simulink model "mOvertakeManeuver"  (R2018b)
settings: Solver=VariableStepAuto  StartTime=0.0  StopTime=simTime  RelTol=1e-3
PreLoadFcn:
  | load 'tableStructure.mat'
InitFcn:
  | modelParams
  | clear markedSmartActorCount;
values from neighbouring files (symbols this model uses):
  initYPos = (scene.RoadNetwork.RoadCenters(1, 2) - laneWidth / 2)    [modelParams.m]
  initYPosRogue = (scene.RoadNetwork.RoadCenters(1, 2) - laneWidth / 2)    [modelParams.m]
  laneWidth = roadWidth / (scene.RoadNetwork.NumMarkings - 1)    [modelParams.m]
  maxLanes = 10    [modelParams.m]
  maxVehicles = 25    [modelParams.m]
  minOvertakeProximity = 50    [modelParams.m]
  numActors = length(scene.vehiclePoses(1).ActorPoses)    [modelParams.m]    (also in sessionLogReader.m = numel(inStruct); visualizer.m = numel(actors))
  numAddedRogueActors = 0    [modelParams.m]
  numLanes = scene.RoadNetwork.NumLanes    [modelParams.m]    (also in sessionLogReader.m = numMarkings-1)
  numSmartActors = 0    [modelParams.m]
  numSmartActorsDM = 0    [modelParams.m]
  rogueActorIdBase = 4000    [modelParams.m]
  safeTimeGap = 1.4    [modelParams.m]
  sensorRange = 600    [modelParams.m]
  smartActors = 0    [modelParams.m]    (also in sessionLogReader.m = repmat(actorPoses(1), [obj.NumSmartActors, 1]))
  smartActorsDM = 0    [modelParams.m]    (also in sessionLogReader.m = repmat(actorPoses(1), [obj.NumSmartActorsDM, 1]))
  standStillGap = 10    [modelParams.m]
  W_SPEC = [Ln1;vdes;vmax;AXadd;AXmult;BXadd;BXmult;EXadd;EXmult;CXconst;CXadd;CXmult;OPDVmult;OPDVadd;BNULLmult;BMAXmult;FAKTORVmult;BMINadd;BMINmult;      RND1n;RND2n;RND3n;RND4n;NRND]    [wiedemannParams.m]
undefined symbols (not defined in the file or in its folder): actorPoseInit, addedRogueVelocity, addedRogueXPosition, DiscIntNeverNeededParam
libraries: dataTableBlockslib x2, mpcadaslib x1
(part 1 of 3)
settings Model: Creator=surongal  LastModifiedBy=surongal
settings DataIOCC: SaveTime=off  ReturnWorkspaceOutputs=on
settings DebuggingCC: InheritedTsInSrcMsg=none
settings SFSimCC: SimUseLocalCustomCode=off
settings RTWCC: RTWUseLocalCustomCode=off

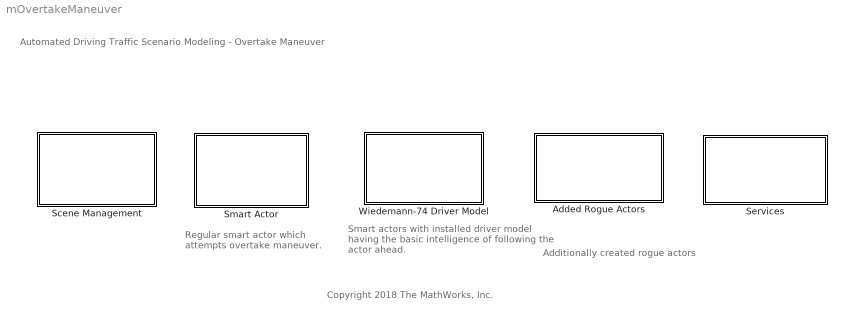
== system mOvertakeManeuver ==
  note: Smart actors with installed driver model having the basic intelligence of following the actor ahead.
  note: Regular smart actor which attempts overtake maneuver.
  note: Copyright 2018 The MathWorks, Inc.
  note: Automated Driving Traffic Scenario Modeling - Overtake Maneuver
  note: Additionally created rogue actors
  Added Rogue Actors : Subsystem  InitFcn=|  mask(Added Rogue Actors){numAddedRogueCars=2, initXPos=[5 550], initXVel=[5 10], rogueActorIdBase=4000}
      | % To get the mask parameter values
      | numAddedRogueActors =str2num( get_param(gcb,'numAddedRogueCars'));
      | addedRogueXPosition = str2num( get_param(gcb,'initXPos'));
      | addedRogueVelocity = str2num( get_param(gcb,'initXVel'));
      | 
      | % To set the mask parameter values
      | set_param(gcb, 'rogueActorIdBase',num2str(rogueActorIdBase));
      mask prompts: numAddedRogueCars "Number of rogue actors"; initXPos "Initial X-position"; initXVel "Initial X-velocity"
      mask help: This block allows to introduce additional rogue actors to the scenario. Each parameter array sequentially contains parameter value for different actors. The scenario should contain only one rogue actors block.
      mask Display:
      | numRogueActors = str2num(get_param(gcb,'numAddedRogueCars'));
      | rogueActorIdBase = str2num(get_param(gcb,'rogueActorIdBase'));
      | disp("Actor IDs : [" + num2str(rogueActorIdBase + [1:numRogueActors]) + "]");
  Scene Management : Subsystem
      mask Display: disp('Scene Management')
  Services : Subsystem
      mask Display: disp('Services');
  Smart Actor : Subsystem  InitFcn=|  mask(Smart Actor){smartActorId=1, aggressivenessLevel=1, maxVelocity=20, maxAcceleration=3, maxDeceleration=-6}
      | smartActorId = str2num(get_param(gcb, 'smartActorId'));
      | % Update the number of actors marked as smart
      | numSmartActors = markedSmartActorCount();
      | 
      | % To keep track of marked smart actors
      | if ismember(smartActorId, smartActors)
      |     error('Actor ID specified is already marked as smart. Mark some other actor ID as smart');
      | else
      |     % To check actorId specified is present or not
      |     if ismember(smartActorId, [actorPoseInit.ActorID])
      |         smartActors(numSmartActors) = smartActorId;
      |     else
      |         error('Actor ID specified in Smart Actor does not exist.');
      |     end
      | end
      | 
      | % To check whether actorId specified as Smart is not already
      | % specified as a smart-actor with driver-model. 
      | driverModelBlockPath = [bdroot, '/Wiedemann-74 Driver Model'];
      | if getSimulinkBlockHandle(driverModelBlockPath) > 0
      |     if strcmp(get_param(driverModelBlockPath, 'commented'), 'off')
      |         % Get Actor IDs with driver model installed
      |         smartIdsDM = str2num(get_param(driverModelBlockPath, 'smartVehIdsDM'));
      |         if sum(ismember(smartActorId, smartIdsDM))
      |             error(['Driver model installation on Smart Actor ' num2str(smartActorId) ' is not supported.']);
      |         end
      |     end
      | end
      | 
      | clear driverModelBlockPath smartIdsDM smartActorId; % clear temporary variables
      mask prompts: smartActorId "ActorID"; aggressivenessLevel "Driver aggressiveness level"; maxVelocity "Max velocity"; maxAcceleration "Max acceleration"; maxDeceleration "Max deceleration"
      mask help: This block allows to mark an actor in the simulation log as a smart actor attempting overtake-maneuver.
      mask init:
      | aggressivenessLevel = str2num(aggressivenessLevel);
      | 
      | % To check whether actorId specified is already
      | % specified in the driver model
      | driverModelBlockPath = [bdroot, '/Wiedemann-74 Driver Model'];
      | if getSimulinkBlockHandle(driverModelBlockPath) > 0
      |     if strcmp(get_param(driverModelBlockPath, 'commented'), 'off')
      |         % Get smart actors with driver model installed
      |         smartIdsDM = str2num(get_param(driverModelBlockPath, 'smartVehIdsDM'));
      |         if sum(ismember(smartActorId, smartIdsDM))
      |             error(['Driver model is already installed on actor with Actor ID : ' num2str(smartActorId) '.']);
      |         end
      |     end
      | end
      mask TypeOptions aggressivenessLevel: 1 | 2 | 3
      mask Display: image('icons/car.png');
  Wiedemann-74 Driver Model : Subsystem  InitFcn=|  mask(Wiedemann-74 Driver Model){smartVehIdsDM=[2], AXAdd=[5], BXMult=[5], vMax=[40], vDes=[30], maxAccel=[4], maxDecel=[-6]}
      | smartActorsDM = str2num( get_param(gcb, 'smartVehIdsDM')); % IDs of vehicles with Driver-Model installed
      | numSmartActorsDM = length(smartActorsDM); % Number of vehicles with Driver-Model installed
      | 
      | wiedemannParams; % Loads Wiedemann model parameters
      | 
      | % All the actors IDs specified for driver-model installation are valid or not
      | if sum(ismember(smartActorsDM, [actorPoseInit.ActorID])) < numSmartActorsDM
      |     error(['Actor IDs [' num2str(smartActorsDM(~ismember(smartActorsDM, [actorPoseInit.ActorID]))) '] specified for driver-model installation does not exist.']);
      | end
      mask prompts: smartVehIdsDM "Vehicles with driver-model"; AXAdd "AXadd (Calibrated parameter affecting desired following distance between stationary vehicles)"; BXMult "BXmult (Calibrated parameter affecting desired minimum following distance at low speed gap)"; vMax "Maximum velocity"; vDes "Desired velocity"; maxAccel "Max acceleration"; maxDecel "Max deceleration"
      mask help: This block allows to install Wiedemann-74 car-follow model on the selected actors. Also, Widemann-74 driver model parameters can be configured for individual cars. Each parameter vector sequentially contains parameter value for different actors in same order as actors are specified in the vehicle's list.
      mask DialogControl maskInfo Prompt: Driver-Model Setup Table
      mask Display: image('icons/carFollow.png');

== system mOvertakeManeuver/Added Rogue Actors ==
  note: Create a set of rogue actors and simulate their movement
  note: Rogue Actors
  "Calculate updated X-Poses " : Subsystem  TreatAsAtomicUnit=on
  Calculate updated Y-Poses : Subsystem  TreatAsAtomicUnit=on
  Get initial poses : MATLAB Function  TreatAsAtomicUnit=on
  Publish to data-table : MATLAB Function  TreatAsAtomicUnit=on
  wires:
  "Calculate updated X-Poses "/2(posVector) -> Publish to data-table/2(xPosVector)
  "Calculate updated X-Poses "/1(velVector) -> Publish to data-table/1(xVelVector)
  Get initial poses/5(yVelocity) -> Calculate updated Y-Poses/2(initVelVector)
  Get initial poses/6(yPosition) -> Calculate updated Y-Poses/3(initPosVector)
  Get initial poses/4(yAcceleration) -> Calculate updated Y-Poses/1(accelVector)
  Calculate updated Y-Poses/1(velVector) -> Publish to data-table/3(yVelVector)
  Calculate updated Y-Poses/2(posVector) -> Publish to data-table/4(yPosVector)
  Get initial poses/1(xAcceleration) -> "Calculate updated X-Poses "/1(accelVector)
  Get initial poses/2(xVelocity) -> "Calculate updated X-Poses "/2(initVelVector)
  Get initial poses/3(xPosition) -> "Calculate updated X-Poses "/3(initPosVector)

== system mOvertakeManeuver/Scene Management ==
  Actor Pose Reader : Subsystem  mask(Actor Pose Reader){ScenarioFileName=scenarioInput, RoadBoundaries=on, LaneBoundaries=on, AllBoundaries=on, LaneMarkings=on, NumLanes=off, NumSmartActorsDM=numSmartActorsDM, NumSmartActors=numSmartActors}
      mask prompts: ScenarioFileName "File name for the recorded scenario:"; RoadBoundaries "Output road boundaries in scenario coordinates"; LaneBoundaries "Output lane boundaries in scenario coordinates"; AllBoundaries "Output all lane boundaries"; LaneMarkings "Output lane markings in scenario coordinates"; NumLanes "Output number of lanes"; NumSmartActorsDM "Number of actors with driver model installed:"; NumSmartActors "Number of actors marked as smart:"
      mask help: The Actor Pose Reader reads actor poses data saved using the drivingScenario record method and road boundary data saved as structs from the drivingScenario roadBoundaries method.
      mask TypeOptions ScenarioFileName: Session Log Reader/ScenarioFileName
      mask TypeOptions RoadBoundaries: Session Log Reader/RoadBoundaries
      mask TypeOptions LaneBoundaries: Session Log Reader/LaneBoundaries
      mask TypeOptions AllBoundaries: Session Log Reader/AllBoundaries
      mask TypeOptions LaneMarkings: Session Log Reader/LaneMarkings
      mask TypeOptions NumLanes: Session Log Reader/NumLanes
      mask TypeOptions NumSmartActorsDM: Session Log Reader/NumSmartActorsDM
      mask TypeOptions NumSmartActors: Session Log Reader/NumSmartActors
      mask Display:
      | disp(['Session Log' char(10) 'Reader']);
      | port_label('output',1,'Actors');
      | port_label('output',2,'Lane Boundaries');
      | port_label('output',3,'Roads');
      | port_label('output',4,'Lane Markings');
  Append poses of added rouge actors for visualization : Subsystem  InitFcn=""
  Publish To Data Table : Subsystem  InitFcn=""
  Visualization : Subsystem  mask(Visualization){XLim=[ -1, 150 ], YLim=[ -30, 30 ], View=Self-Centered view, NumSmartActors=numSmartActors, HasActors=on, HasRoads=on, HasLaneMarkings=on}
      mask prompts: XLim "Minimum and maximum distance in the longitudinal axis:"; YLim "Minimum and maximum distance in the lateral axis:"; View "Visualization type:"; NumSmartActors "Number of smart actors:"; HasActors "Display actors data"; HasRoads "Display road boundary data"; HasLaneMarkings "Display lane markings"
      mask help: The Visualization block creates and maintains a bird's-eye plot. You can opt for 'World-coordinate' view or 'Self-centered' view.
      mask TypeOptions XLim: Visualization/XLim
      mask TypeOptions YLim: Visualization/YLim
      mask TypeOptions View: Visualization/View
      mask TypeOptions NumSmartActors: Visualization/NumSmartActors
      mask TypeOptions HasActors: Visualization/HasActors
      mask TypeOptions HasRoads: Visualization/HasRoads
      mask TypeOptions HasLaneMarkings: Visualization/HasLaneMarkings
      mask Display:
      | disp('Visualizer');
      | port_label('input',1,'Actors');
      | port_label('input',2,'Roads');
      | port_label('input',3,'Lane Markings');
  wires:
  Actor Pose Reader/3(Roads) -> Visualization/2(Roads)
  Actor Pose Reader/1(Actors) -> Publish To Data Table/1(Actors), Append poses of added rouge actors for visualization/1(simulationLogActors)
  Actor Pose Reader/2(Lane Boundaries) -> Publish To Data Table/2(Lane Boundaries)
  Actor Pose Reader/4(Lane Markings) -> Visualization/3(Lane Markings)
  Append poses of added rouge actors for visualization/1(actors) -> Visualization/1(Actors)  "actorPoses"

== system mOvertakeManeuver/Services ==
  note: Queries used by Smart Agents
  "Actor-Pose " : dataTableBlockslib/Data Table Service  tableName=Actor  tableSize=30  tableFormat=Vehicle  tableQueries={{OvertakeQueries.VehiclesAheadSameLane,'findVehiclesAheadSameLane'},{OvertakeQueries.VehiclesAheadLeftLane,'findVehiclesAheadLeftLane'}}  mask(DataTableService){}
      mask Display: disp('Actor Pose Information');
  Find approaching vehicles in the left lane : Subsystem  TreatAsAtomicUnit=on
  Find vehicles ahead in the same lane : Subsystem  TreatAsAtomicUnit=on
  Global to self-centered pose conversion : Subsystem  TreatAsAtomicUnit=on
  "Scene " : dataTableBlockslib/Data Table Service  tableName=Scenario  tableSize=30  tableFormat=LaneBoundaries  tableQueries={}  mask(DataTableService){}
      mask Display: disp('Scene Information');

== system mOvertakeManeuver/Smart Actor ==
  note: This subsystem simulates an actor which is nominated as a smart actor,
      | among the actors present in input driving session log. The primary intelligence in this
      | smart actor is to overtake, if environment around it allows for it.
  note: Nominated Smart Actor
  Load Initial Pose : MATLAB Function  TreatAsAtomicUnit=on
  Smart Actor system : Subsystem
  Write pose to Data-Table : MATLAB Function  TreatAsAtomicUnit=on
  wires:
  Smart Actor system/1(Updated Pose) -> Write pose to Data-Table/1(pose)
  Load Initial Pose/1(initPose) -> Smart Actor system/1(Initial Pose)

== system mOvertakeManeuver/Wiedemann-74 Driver Model ==
  note: Apply driver-model on selected actors:
      | Calculated updated driver-model-governed poses and write into data-table.
  Apply driver-model : Subsystem
  Get Follow and Lead car : MATLAB Function  TreatAsAtomicUnit=on
  Gets the vehicles ahead in sorted order of the distance from this actor. : Subsystem  TreatAsAtomicUnit=on
  Simulation Time : DigitalClock  SampleTime=-1
  Write smart-actor poses in data-table : MATLAB Function  TreatAsAtomicUnit=on
  wires:
  Apply driver-model/1(velVector) -> Write smart-actor poses in data-table/1(velVector)
  Get Follow and Lead car/5(leadAcc) -> Apply driver-model/5(leadVehAcc)
  Get Follow and Lead car/4(leadVel) -> Apply driver-model/4(leadVehSpd)
  Apply driver-model/2(posVector) -> Write smart-actor poses in data-table/2(posVector)
  Get Follow and Lead car/2(follVel) -> Apply driver-model/2(smartVehSpd)
  Simulation Time/1 -> Get Follow and Lead car/1(timestamp)
  Get Follow and Lead car/1(follPos) -> Apply driver-model/1(smartVehPos)
  Get Follow and Lead car/3(leadPos) -> Apply driver-model/3(leadVehPos)

== system mOvertakeManeuver/Added Rogue Actors/Calculate updated X-Poses  ==
  accelVector : Inport  Partition=on  PartitionDimension=1  PartitionWidth=1  PartitionOffset=0
  initVelVector : Inport  Port=2  Partition=on  PartitionDimension=1  PartitionWidth=1  PartitionOffset=0
  initPosVector : Inport  Port=3  Partition=on  PartitionDimension=1  PartitionWidth=1  PartitionOffset=0
  For Each : ForEach  DisableCoverage=on  IndexMode=One-based
  Update Poses : Subsystem
  velVector : Outport  ConcatenationDimension=1
  posVector : Outport  Port=2  ConcatenationDimension=1
  wires:
  accelVector/1 -> Update Poses/1(accVector)
  initPosVector/1 -> Update Poses/3(initPosVector)
  initVelVector/1 -> Update Poses/2(initVelVector)
  Update Poses/2(Out2) -> posVector/1
  Update Poses/1(Out1) -> velVector/1

== system mOvertakeManeuver/Added Rogue Actors/Calculate updated Y-Poses ==
  accelVector : Inport  Partition=on  PartitionDimension=1  PartitionWidth=1  PartitionOffset=0
  initVelVector : Inport  Port=2  Partition=on  PartitionDimension=1  PartitionWidth=1  PartitionOffset=0
  initPosVector : Inport  Port=3  Partition=on  PartitionDimension=1  PartitionWidth=1  PartitionOffset=0
  For Each : ForEach  DisableCoverage=on  IndexMode=One-based
  Update Poses : Subsystem
  velVector : Outport  ConcatenationDimension=1
  posVector : Outport  Port=2  ConcatenationDimension=1
  wires:
  Update Poses/1(Out1) -> velVector/1
  Update Poses/2(Out2) -> posVector/1
  initVelVector/1 -> Update Poses/2(initVelVector)
  initPosVector/1 -> Update Poses/3(initPosVector)
  accelVector/1 -> Update Poses/1(accVector)

== system mOvertakeManeuver/Scene Management/Actor Pose Reader ==
  Read smart actor poses : MATLAB Function  TreatAsAtomicUnit=on
  Session Log Reader : MATLABSystem  System=sessionLogReader  ScenarioFileName=scenarioInput  NumSmartActorsDM=NumSmartActorsDM  NumSmartActors=NumSmartActors  SmartActorSource=Input port  SmartActorID=1  RoadBoundaries=on  LaneBoundaries=on  AllBoundaries=on  LaneBoundaryDistance=0:0.5:9.5  LaneBoundaryLocation=center  NumLanes=off  LaneMarkings=on  BusNameSource=Auto  BusName2Source=Auto  BusName3Source=Auto  SimulateUsing=Interpreted execution
      mask Type: sessionLogReader
      mask Display:
      | disp(['Session Log' char(10) 'Reader']);
      | port_label('input',1,'actors');
      | port_label('output',1,'Actors');
      | port_label('output',2,'Roads');
      | port_label('output',3,'Lane Boundaries');
      | port_label('output',4,'Lane Markings');
  Actors : Outport
  Lane Boundaries : Outport  Port=2
  Roads : Outport  Port=3
  Lane Markings : Outport  Port=4
  wires:
  Session Log Reader/1 -> Actors/1
  Session Log Reader/2 -> Roads/1
  Session Log Reader/4 -> Lane Markings/1
  Session Log Reader/3 -> Lane Boundaries/1
  Read smart actor poses/1(actorPoses) -> Session Log Reader/1

== system mOvertakeManeuver/Scene Management/Append poses of added rouge actors for visualization ==
  simulationLogActors : Inport
  Appending Rouge Actor Poses : MATLAB Function  TreatAsAtomicUnit=on
  Bus Selector1 : BusSelector  OutputSignals=Actors
  actors : Outport
  wires:
  Bus Selector1/1 -> Appending Rouge Actor Poses/1(simulationLogActors)  "<Actors>"
  simulationLogActors/1 -> Bus Selector1/1
  Appending Rouge Actor Poses/1(Actors) -> actors/1

== system mOvertakeManeuver/Scene Management/Publish To Data Table ==
  Actors : Inport
  Lane Boundaries : Inport  Port=2
  Bus Selector : BusSelector  OutputSignals=Actors
  Write inital pose from session-logs into data-table : MATLAB Function  Priority=0  TreatAsAtomicUnit=on
      settings: AttributesFormatString=Pri = %<Priority>
  update data tables : MATLAB Function  TreatAsAtomicUnit=on
  wires:
  Actors/1 -> Bus Selector/1
  Bus Selector/1 -> update data tables/1(actors)  "<Actors>"
  Lane Boundaries/1 -> update data tables/2(laneBoundaryInfo)

== system mOvertakeManeuver/Scene Management/Visualization ==
  Actors : Inport
  Roads : Inport  Port=2
  Lane Markings : Inport  Port=3
  Visualization : MATLABSystem  StartFcn=|  StopFcn=""  System=visualizer  XLim=XLim  YLim=YLim  NumSmartActors=NumSmartActors  View=Self-Centered view  smartActorIndex=1  HasActors=on  HasRoads=on  HasLaneMarkings=on
      | % checks whether the view is set to Ego Centric View
      | if strcmp(get_param(gcb, 'View'), 'Self-Centered view')
      |     % checks whether to populate the list modal dialog
      |     if numSmartActors > 1
      |         List = repmat("Added Ego (Actor ID : ", [numSmartActors 1]);
      |         for n = 1 : numSmartActors
      |             List(n, 1) =   "Nominated Ego  (Actor ID : "+smartActors(n)+")";
      |         end
      |         
      |         [indx, isSelected] = listdlg('PromptString', 'Select the ego actor ', 'ListString', List, 'SelectionMode', 'single', 'InitialValue', 1);
      |         % if user closes the dialog without selecting from list
      |         if isSelected == 0
      |             % set the indx to 1
      |             indx = 1;
      |         end
      |     else
      |         indx = 1;
      |     end
      |     
      |     % Set the mask parameters
      |     set_param(gcb, 'smartActorIndex', num2str(indx));
      | end
      | 
      | clear List n indx isSelected; % clears temporary variables
      mask Type: visualizer
      mask Display:
      | disp('Visualizer');
      | port_label('input',1,'Actors');
      | port_label('input',2,'Roads');
      | port_label('input',3,'Lane Markings');
  wires:
  Roads/1 -> Visualization/2
  Lane Markings/1 -> Visualization/3
  Actors/1 -> Visualization/1

== system mOvertakeManeuver/Services/Find approaching vehicles in the left lane ==
  findVehiclesAheadLeftLane : TriggerPort  TriggerType=function-call  IsSimulinkFunction=on  FunctionName=findVehiclesAheadLeftLane  FunctionVisibility=scoped  VariantControl=(inherit)
  MATLAB Function : MATLAB Function  TreatAsAtomicUnit=on
  refEntry : ArgIn  OutDataTypeStr=Bus: Vehicle  ArgumentName=refEntry
  otherEntry : ArgIn  Port=2  OutDataTypeStr=Bus: Vehicle  ArgumentName=otherEntry
  matched : ArgOut  DisableCoverage=on  OutDataTypeStr=boolean  ArgumentName=matched
  wires:
  MATLAB Function/1(matched) -> matched/1
  refEntry/1 -> MATLAB Function/1(refPose)
  otherEntry/1 -> MATLAB Function/2(candidatePose)

== system mOvertakeManeuver/Services/Find vehicles ahead in the same lane ==
  findVehiclesAheadSameLane : TriggerPort  TriggerType=function-call  IsSimulinkFunction=on  FunctionName=findVehiclesAheadSameLane  FunctionVisibility=scoped  VariantControl=(inherit)
  MATLAB Function : MATLAB Function  TreatAsAtomicUnit=on
  refEntry : ArgIn  OutDataTypeStr=Bus: Vehicle  ArgumentName=refEntry
  otherEntry : ArgIn  Port=2  OutDataTypeStr=Bus: Vehicle  ArgumentName=otherEntry
  matched : ArgOut  DisableCoverage=on  OutDataTypeStr=boolean  ArgumentName=matched
  wires:
  MATLAB Function/1(matched) -> matched/1
  refEntry/1 -> MATLAB Function/1(refPose)
  otherEntry/1 -> MATLAB Function/2(candidatePose)

== system mOvertakeManeuver/Services/Global to self-centered pose conversion ==
  globalToSelfCentered : TriggerPort  TriggerType=function-call  IsSimulinkFunction=on  FunctionName=globalToSelfCentered  VariantControl=(inherit)
  Self-Centered Pose Conversion : MATLAB Function  TreatAsAtomicUnit=on
  refEntry : ArgIn  DisableCoverage=on  OutDataTypeStr=Bus: Vehicle  ArgumentName=refEntry
  otherEntry : ArgIn  Port=2  OutDataTypeStr=Bus: Vehicle  ArgumentName=otherEntry
  selfRefInfo : ArgOut  DisableCoverage=on  OutDataTypeStr=Bus: Vehicle  ArgumentName=selfRefInfo
  wires:
  refEntry/1 -> Self-Centered Pose Conversion/1(selfPose)
  otherEntry/1 -> Self-Centered Pose Conversion/2(otherVehPose)
  Self-Centered Pose Conversion/1(egoCentricInfo) -> selfRefInfo/1

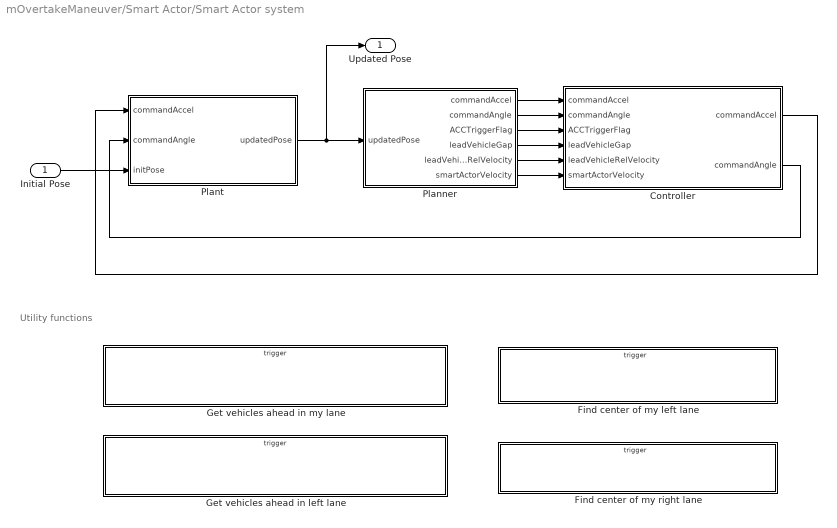
== system mOvertakeManeuver/Smart Actor/Smart Actor system ==
  note: Utility functions
  Initial Pose : Inport
  Controller : Subsystem
  Find center of my left lane : Subsystem  TreatAsAtomicUnit=on
  Find center of my right lane : Subsystem  TreatAsAtomicUnit=on
  Get vehicles ahead in left lane : Subsystem  TreatAsAtomicUnit=on
  Get vehicles ahead in my lane : Subsystem  TreatAsAtomicUnit=on
  Planner : Subsystem
  Plant : Subsystem
  Updated Pose : Outport
  wires:
  Initial Pose/1 -> Plant/3(initPose)
  Controller/1(commandAccel) -> Plant/1(" commandAccel")
  Plant/1(updatedPose) -> Planner/1(updatedPose), Updated Pose/1
  Planner/1(commandAccel) -> Controller/1(" commandAccel")
  Planner/2(commandAngle) -> Controller/2(" commandAngle")
  Planner/3(ACCTriggerFlag) -> Controller/3(ACCTriggerFlag)
  Planner/4(leadVehicleGap) -> Controller/4(" leadVehicleGap")
  Planner/5(leadVehicleRelVelocity) -> Controller/5(" leadVehicleRelVelocity")
  Planner/6(smartActorVelocity) -> Controller/6(" smartActorVelocity")
  Controller/2(commandAngle) -> Plant/2(commandAngle)

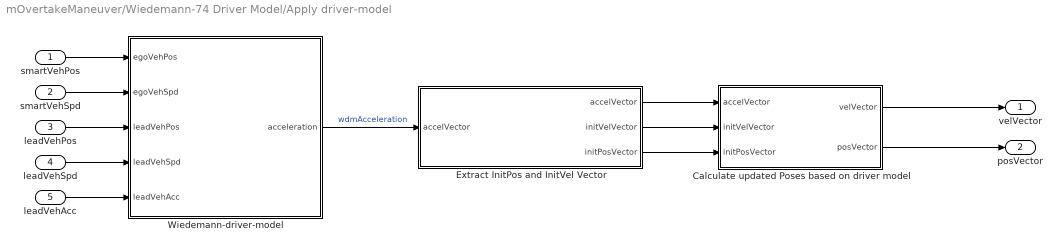
== system mOvertakeManeuver/Wiedemann-74 Driver Model/Apply driver-model ==
  smartVehPos : Inport
  smartVehSpd : Inport  Port=2
  leadVehPos : Inport  Port=3
  leadVehSpd : Inport  Port=4
  leadVehAcc : Inport  Port=5
  Calculate updated Poses based on driver model : Subsystem  TreatAsAtomicUnit=on
  Extract InitPos and InitVel Vector : MATLAB Function  TreatAsAtomicUnit=on
  Wiedemann-driver-model : Subsystem
  velVector : Outport
  posVector : Outport  Port=2
  wires:
  smartVehPos/1 -> Wiedemann-driver-model/1(egoVehPos)
  smartVehSpd/1 -> Wiedemann-driver-model/2(egoVehSpd)
  leadVehPos/1 -> Wiedemann-driver-model/3(leadVehPos)
  leadVehSpd/1 -> Wiedemann-driver-model/4(leadVehSpd)
  leadVehAcc/1 -> Wiedemann-driver-model/5(leadVehAcc)
  Calculate updated Poses based on driver model/1(velVector) -> velVector/1
  Calculate updated Poses based on driver model/2(posVector) -> posVector/1
  Extract InitPos and InitVel Vector/1(accelVector) -> Calculate updated Poses based on driver model/1(accelVector)
  Extract InitPos and InitVel Vector/3(initPosVector) -> Calculate updated Poses based on driver model/3(initPosVector)
  Extract InitPos and InitVel Vector/2(initVelVector) -> Calculate updated Poses based on driver model/2(initVelVector)
  Wiedemann-driver-model/1(acceleration) -> Extract InitPos and InitVel Vector/1("accelVector ")  "wdmAcceleration"

== system mOvertakeManeuver/Wiedemann-74 Driver Model/Gets the vehicles ahead in sorted order of the distance from this actor. ==
  getVehAheadSorted : TriggerPort  TriggerType=function-call  IsSimulinkFunction=on  FunctionName=getVehAheadSorted  FunctionVisibility=scoped  VariantControl=(inherit)
  Gets the vehicles ahead in sorted order of the gap : MATLAB Function  TreatAsAtomicUnit=on
  actorId : ArgIn  DisableCoverage=on  ArgumentName=actorId
  numVeh : ArgOut  ArgumentName=numVeh
  vehAheadInfo : ArgOut  Port=2  OutDataTypeStr=Bus: Vehicle  PortDimensions=maxVehicles  ArgumentName=vehAheadInfo
  wires:
  actorId/1 -> Gets the vehicles ahead in sorted order of the gap/1(actorId)
  Gets the vehicles ahead in sorted order of the gap/1(vehAheadInfo) -> vehAheadInfo/1
  Gets the vehicles ahead in sorted order of the gap/2(numVeh) -> numVeh/1

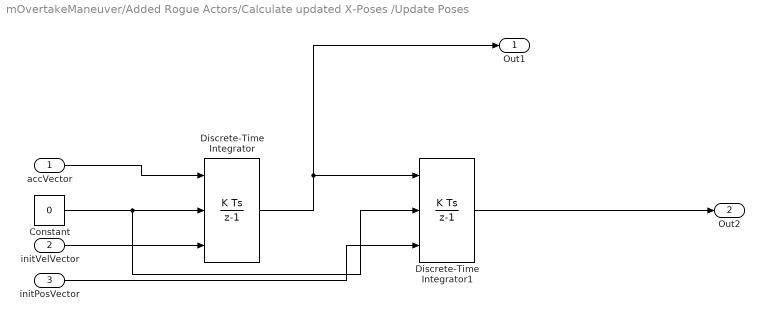
== system mOvertakeManeuver/Added Rogue Actors/Calculate updated X-Poses /Update Poses ==
  accVector : Inport
  initVelVector : Inport  Port=2
  initPosVector : Inport  Port=3
  Constant : Constant  Value=0
  Discrete-Time Integrator : DiscreteIntegrator  ExternalReset=level  InitialConditionSource=external  SampleTime=-1  ICPrevOutput=DiscIntNeverNeededParam  ICPrevScaledInput=DiscIntNeverNeededParam
  Discrete-Time Integrator1 : DiscreteIntegrator  ExternalReset=level  InitialConditionSource=external  SampleTime=-1  ICPrevOutput=DiscIntNeverNeededParam  ICPrevScaledInput=DiscIntNeverNeededParam
  Out1 : Outport
  Out2 : Outport  Port=2
  wires:
  Discrete-Time Integrator/1 -> Discrete-Time Integrator1/1, Out1/1
  accVector/1 -> Discrete-Time Integrator/1
  Discrete-Time Integrator1/1 -> Out2/1
  initPosVector/1 -> Discrete-Time Integrator1/3
  Constant/1 -> Discrete-Time Integrator1/2, Discrete-Time Integrator/2
  initVelVector/1 -> Discrete-Time Integrator/3

== system mOvertakeManeuver/Added Rogue Actors/Calculate updated Y-Poses/Update Poses ==
  accVector : Inport
  initVelVector : Inport  Port=2
  initPosVector : Inport  Port=3
  Constant : Constant  Value=0
  Discrete-Time Integrator : DiscreteIntegrator  ExternalReset=level  InitialConditionSource=external  SampleTime=-1  ICPrevOutput=DiscIntNeverNeededParam  ICPrevScaledInput=DiscIntNeverNeededParam
  Discrete-Time Integrator1 : DiscreteIntegrator  ExternalReset=level  InitialConditionSource=external  SampleTime=-1  ICPrevOutput=DiscIntNeverNeededParam  ICPrevScaledInput=DiscIntNeverNeededParam
  Out1 : Outport
  Out2 : Outport  Port=2
  wires:
  Constant/1 -> Discrete-Time Integrator1/2, Discrete-Time Integrator/2
  initPosVector/1 -> Discrete-Time Integrator1/3
  Discrete-Time Integrator1/1 -> Out2/1
  accVector/1 -> Discrete-Time Integrator/1
  initVelVector/1 -> Discrete-Time Integrator/3
  Discrete-Time Integrator/1 -> Discrete-Time Integrator1/1, Out1/1

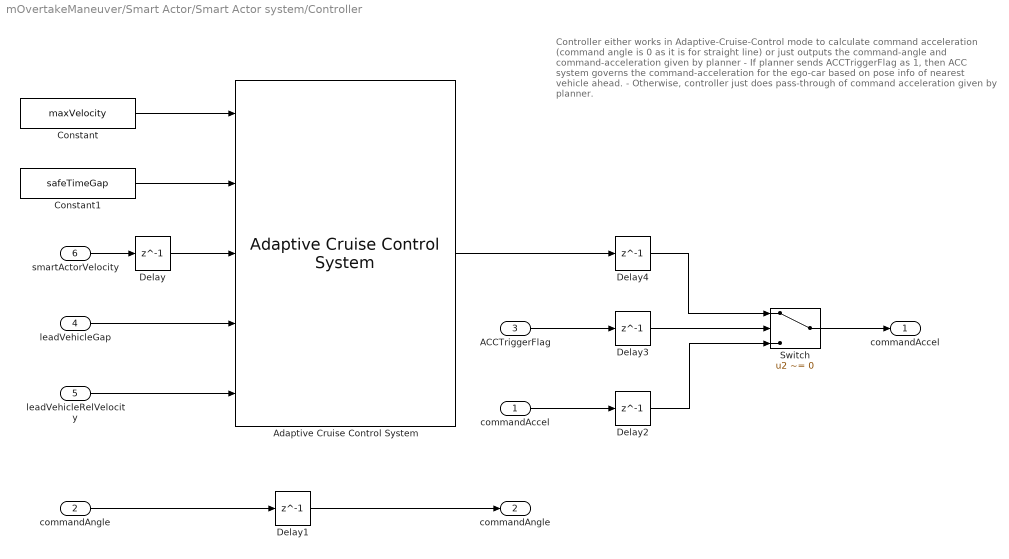
== system mOvertakeManeuver/Smart Actor/Smart Actor system/Controller ==
  note: Controller either works in Adaptive-Cruise-Control mode to calculate
      | command acceleration (command angle is 0 as it is for straight line) or
      | just outputs the command-angle and command-acceleration given by
      | planner
      | - If planner sends ACCTriggerFlag as 1, then ACC system governs the
      |   command-acceleration for the ego-car based on pose info
      |   of nearest vehicle ahead.
      | - Otherwise, controller just does pass-through of command acceleration
      |   given by planner.
  " commandAccel" : Inport
  " commandAngle" : Inport  Port=2
  ACCTriggerFlag : Inport  Port=3
  " leadVehicleGap" : Inport  Port=4
  " leadVehicleRelVelocity" : Inport  Port=5
  " smartActorVelocity" : Inport  Port=6
  Adaptive Cruise Control System : mpcadaslib/Adaptive Cruise Control System  EgoModel=tf(1,[0.5,1,0])  InitialEgoVelocity=abs(actorPoseInit(smartActorId).Velocity(1))  DefaultSpacing=standStillGap  MaxVelocity=maxVelocity  MinAcceleration=maxDeceleration  amin_ext=off  MaxAcceleration=maxAcceleration  amax_ext=off  Ts=0.1  PredictionHorizon=30  ControllerBehavior=0.5  suboptimal=off  maxiter=10  datatypeopt=double  optmode=off  trackmode=off
      settings: SourceProductName=Model Predictive Control Toolbox
  Constant : Constant  Value=maxVelocity  SampleTime=-1
  Constant1 : Constant  Value=safeTimeGap
  Delay{,1..4} (5 alike) : Delay  DelayLength=1  InitialCondition=0
  Switch : Switch  Criteria=u2 ~= 0
  commandAccel : Outport
  commandAngle : Outport  Port=2
  wires:
  " commandAccel"/1 -> Delay2/1
  Constant/1 -> Adaptive Cruise Control System/1
  " leadVehicleGap"/1 -> Adaptive Cruise Control System/4
  " leadVehicleRelVelocity"/1 -> Adaptive Cruise Control System/5
  " commandAngle"/1 -> Delay1/1
  Delay/1 -> Adaptive Cruise Control System/3
  Delay1/1 -> commandAngle/1
  " smartActorVelocity"/1 -> Delay/1
  ACCTriggerFlag/1 -> Delay3/1
  Delay2/1 -> Switch/3
  Delay3/1 -> Switch/2
  Delay4/1 -> Switch/1
  Adaptive Cruise Control System/1 -> Delay4/1
  Constant1/1 -> Adaptive Cruise Control System/2
  Switch/1 -> commandAccel/1

== system mOvertakeManeuver/Smart Actor/Smart Actor system/Find center of my left lane ==
  getLeftLane : TriggerPort  TriggerType=function-call  IsSimulinkFunction=on  FunctionName=getLeftLane  FunctionVisibility=scoped  VariantControl=(inherit)
  Get left lane center Y : MATLAB Function  TreatAsAtomicUnit=on
  currPose : ArgIn  OutDataTypeStr=Bus: Vehicle  ArgumentName=currPose
  leftLaneCenter : ArgOut  ArgumentName=leftLaneCenter
  wires:
  currPose/1 -> Get left lane center Y/1(currPose)
  Get left lane center Y/1(leftlaneY) -> leftLaneCenter/1

== system mOvertakeManeuver/Smart Actor/Smart Actor system/Find center of my right lane ==
  getRightLane : TriggerPort  TriggerType=function-call  IsSimulinkFunction=on  FunctionName=getRightLane  FunctionVisibility=scoped  VariantControl=(inherit)
  Get right lane center Y : MATLAB Function  TreatAsAtomicUnit=on
  currPose : ArgIn  OutDataTypeStr=Bus: Vehicle  ArgumentName=currPose
  rightLaneCenter : ArgOut  ArgumentName=rightLaneCenter
  wires:
  Get right lane center Y/1(rightLaneY) -> rightLaneCenter/1
  currPose/1 -> Get right lane center Y/1(currPose)

== system mOvertakeManeuver/Smart Actor/Smart Actor system/Get vehicles ahead in left lane ==
  getVehAheadLeftLaneSorted : TriggerPort  TriggerType=function-call  IsSimulinkFunction=on  FunctionName=getVehAheadLeftLaneSorted  FunctionVisibility=scoped  VariantControl=(inherit)
  Get vehicles ahead in left lane : MATLAB Function  TreatAsAtomicUnit=on
  currPose : ArgIn  OutDataTypeStr=Bus: Vehicle  ArgumentName=currPose
  numVeh : ArgOut  ArgumentName=numVeh
  vehAheadInfo : ArgOut  Port=2  OutDataTypeStr=Bus: Vehicle  PortDimensions=maxVehicles  ArgumentName=vehAheadInfo
  wires:
  Get vehicles ahead in left lane/1(vehAheadInfo) -> vehAheadInfo/1
  Get vehicles ahead in left lane/2(numVeh) -> numVeh/1
  currPose/1 -> Get vehicles ahead in left lane/1(currPose)

== system mOvertakeManeuver/Smart Actor/Smart Actor system/Get vehicles ahead in my lane ==
  getVehAheadSameLaneSorted : TriggerPort  TriggerType=function-call  IsSimulinkFunction=on  FunctionName=getVehAheadSameLaneSorted  FunctionVisibility=scoped  VariantControl=(inherit)
  Get vehicles ahead in my lane : MATLAB Function  TreatAsAtomicUnit=on
  currPose : ArgIn  OutDataTypeStr=Bus: Vehicle  ArgumentName=currPose
  numVeh : ArgOut  ArgumentName=numVeh
  vehAheadInfo : ArgOut  Port=2  OutDataTypeStr=Bus: Vehicle  PortDimensions=maxVehicles  ArgumentName=vehAheadInfo
  wires:
  Get vehicles ahead in my lane/1(vehAheadInfo) -> vehAheadInfo/1
  Get vehicles ahead in my lane/2(numVeh) -> numVeh/1
  currPose/1 -> Get vehicles ahead in my lane/1(currPose)

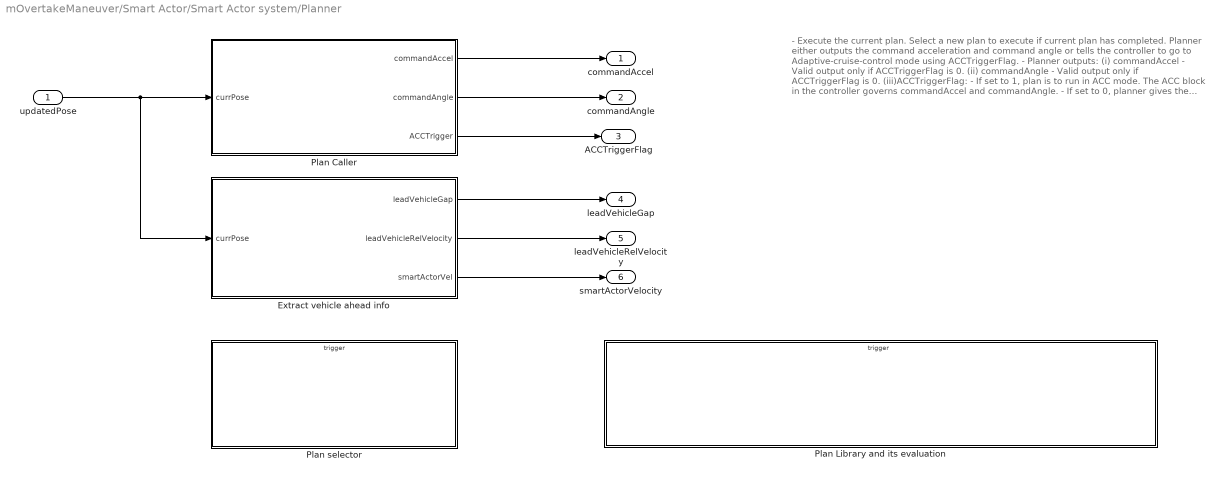
== system mOvertakeManeuver/Smart Actor/Smart Actor system/Planner ==
  note: - Execute the current plan. Select a new plan to execute if
      | current plan has completed. Planner either outputs the command
      | acceleration and command angle or tells the controller to go to
      | Adaptive-cruise-control mode using ACCTriggerFlag.
      |
      | - Planner outputs:
      | (i) commandAccel -  Valid output only if ACCTriggerFlag is 0.
      | (ii) commandAngle - Valid output only if ACCTriggerFlag is 0.
      | (iii)ACCTriggerFlag:
      |        - If set to 1, plan is to run in ACC mode. The ACC block in the
      |          controller governs commandAccel and commandAngle.
      |        - If set to 0, planner gives the commandAccel and commandAngle.
      | (iv) Other 3 outputs (leadVehicleGap, leadVehicleRelVelocity,
      |       smartActorVelocity) are the required inputs for ACC controlled
      |       movement and controller uses them only if ACCTriggerFlag = 1
  updatedPose : Inport
  Extract vehicle ahead info : MATLAB Function  TreatAsAtomicUnit=on
  Plan Caller : MATLAB Function  TreatAsAtomicUnit=on
  Plan Library and its evaluation : Subsystem  TreatAsAtomicUnit=on
  Plan selector : Subsystem  TreatAsAtomicUnit=on
  commandAccel : Outport
  commandAngle : Outport  Port=2
  ACCTriggerFlag : Outport  Port=3
  leadVehicleGap : Outport  Port=4
  leadVehicleRelVelocity : Outport  Port=5
  smartActorVelocity : Outport  Port=6
  wires:
  updatedPose/1 -> Extract vehicle ahead info/1(currPose), Plan Caller/1(currPose)
  Plan Caller/1(commandAccel) -> commandAccel/1
  Plan Caller/2(commandAngle) -> commandAngle/1
  Extract vehicle ahead info/2(leadVehicleRelVelocity) -> leadVehicleRelVelocity/1
  Extract vehicle ahead info/1(leadVehicleGap) -> leadVehicleGap/1
  Extract vehicle ahead info/3(smartActorVel) -> smartActorVelocity/1
  Plan Caller/3(ACCTrigger) -> ACCTriggerFlag/1

== system mOvertakeManeuver/Smart Actor/Smart Actor system/Plant ==
  note: Update the position of smart actor based on controller outputs
      |  (command angle and command acceleration).
  " commandAccel" : Inport
  commandAngle : Inport  Port=2
  initPose : Inport  Port=3
  Smart actor movement : MATLAB Function  TreatAsAtomicUnit=on
  X-movement : Subsystem  TreatAsAtomicUnit=on
  Y-movement : Subsystem  TreatAsAtomicUnit=on
  updatedPose : Outport
  wires:
  initPose/1 -> Smart actor movement/3(initPose)
  Smart actor movement/1(updatedPose) -> updatedPose/1
  " commandAccel"/1 -> Smart actor movement/1(commandAccel)
  commandAngle/1 -> Smart actor movement/2(commandAngle)

== system mOvertakeManeuver/Wiedemann-74 Driver Model/Apply driver-model/Calculate updated Poses based on driver model ==
  accelVector : Inport  Partition=on  PartitionDimension=1  PartitionWidth=1  PartitionOffset=0
  initVelVector : Inport  Port=2  Partition=on  PartitionDimension=1  PartitionWidth=1  PartitionOffset=0
  initPosVector : Inport  Port=3  Partition=on  PartitionDimension=1  PartitionWidth=1  PartitionOffset=0
  For Each : ForEach  DisableCoverage=on  IndexMode=One-based
  Update Poses : Subsystem
  velVector : Outport  ConcatenationDimension=1
  posVector : Outport  Port=2  ConcatenationDimension=1
  wires:
  accelVector/1 -> Update Poses/1(accVector)
  initPosVector/1 -> Update Poses/3(initPosVector)
  initVelVector/1 -> Update Poses/2(initVelVector)
  Update Poses/2(Out2) -> posVector/1
  Update Poses/1(Out1) -> velVector/1

== system mOvertakeManeuver/Wiedemann-74 Driver Model/Apply driver-model/Wiedemann-driver-model ==
  egoVehPos : Inport
  egoVehSpd : Inport  Port=2
  leadVehPos : Inport  Port=3
  leadVehSpd : Inport  Port=4
  leadVehAcc : Inport  Port=5
  Apply Transfer Function : Subsystem  TreatAsAtomicUnit=on
  Judgement : Subsystem
  acceleration : Outport
  wires:
  Apply Transfer Function/1(Out1) -> acceleration/1
  Judgement/1(egoAccCmd) -> Apply Transfer Function/1(egoAccCmd)
  egoVehSpd/1 -> Judgement/2(egoVehSpd)
  egoVehPos/1 -> Judgement/1(egoVehPos)
  leadVehAcc/1 -> Judgement/5(leadVehAcc)
  leadVehSpd/1 -> Judgement/4(leadVehSpd)
  leadVehPos/1 -> Judgement/3(leadVehPos)

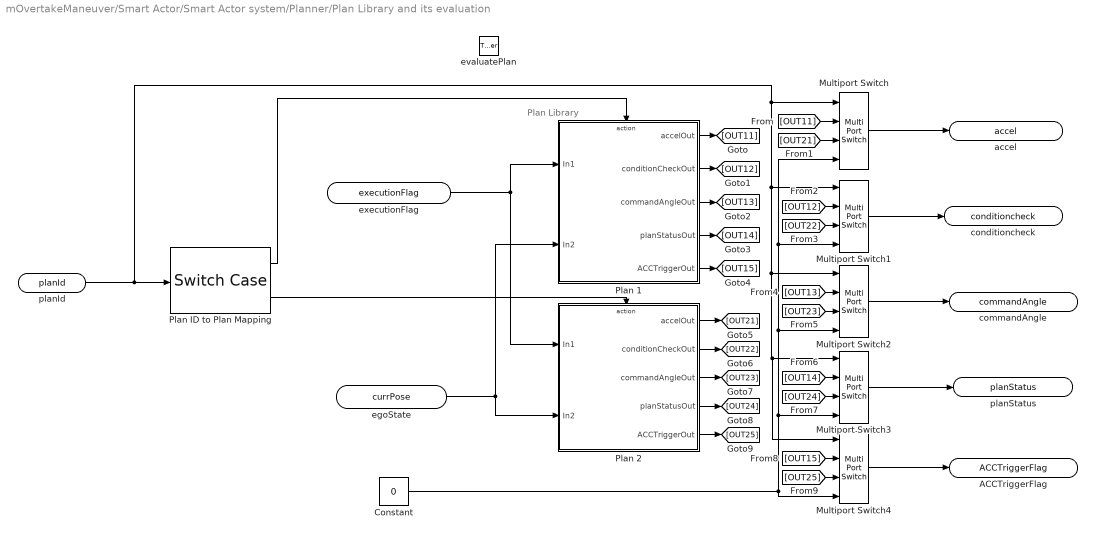
== system mOvertakeManeuver/Smart Actor/Smart Actor system/Planner/Plan Library and its evaluation ==
  note: Plan Library
  evaluatePlan : TriggerPort  TriggerType=function-call  IsSimulinkFunction=on  FunctionName=evaluatePlan  FunctionVisibility=scoped  VariantControl=(inherit)
  Constant : Constant  Value=0  SampleTime=-1
  Multiport Switch{,1..4} (5 alike) : MultiPortSwitch  Inputs=2  DataPortForDefault=Additional data port
  Plan 1 : Subsystem  TreatAsAtomicUnit=on
  Plan 2 : Subsystem  TreatAsAtomicUnit=on
  Plan ID to Plan Mapping : SwitchCase  CaseConditions={1,2}  ShowDefaultCase=off
  planId : ArgIn  DisableCoverage=on  ArgumentName=planId
  executionFlag : ArgIn  Port=2  ArgumentName=executionFlag
  egoState : ArgIn  Port=3  OutDataTypeStr=Bus: Vehicle  ArgumentName=currPose
  accel : ArgOut  DisableCoverage=on  ArgumentName=accel
  conditioncheck : ArgOut  DisableCoverage=on  Port=2  ArgumentName=conditioncheck
  commandAngle : ArgOut  DisableCoverage=on  Port=3  ArgumentName=commandAngle
  planStatus : ArgOut  DisableCoverage=on  Port=4  ArgumentName=planStatus
  ACCTriggerFlag : ArgOut  DisableCoverage=on  Port=5  ArgumentName=ACCTriggerFlag
  wires:
  Plan ID to Plan Mapping/2 -> Plan 2/Action
  Plan ID to Plan Mapping/1 -> Plan 1/Action
  executionFlag/1 -> Plan 2/1(In1), Plan 1/1(In1)
  planId/1 -> Multiport Switch4/1, Multiport Switch3/1, Multiport Switch2/1, Multiport Switch1/1, Multiport Switch/1, Plan ID to Plan Mapping/1
  egoState/1 -> Plan 1/2(In2), Plan 2/2(In2)
  Constant/1 -> Multiport Switch1/4, Multiport Switch/4, Multiport Switch2/4, Multiport Switch3/4, Multiport Switch4/4
  Multiport Switch/1 -> accel/1
  Multiport Switch2/1 -> commandAngle/1
  Multiport Switch1/1 -> conditioncheck/1
  Multiport Switch3/1 -> planStatus/1
  Multiport Switch4/1 -> ACCTriggerFlag/1
  Plan 1/1(accelOut) -> [OUT11]
  Plan 1/2(conditionCheckOut) -> [OUT12]
  Plan 1/3(commandAngleOut) -> [OUT13]
  Plan 1/4(planStatusOut) -> [OUT14]
  Plan 1/5(ACCTriggerOut) -> [OUT15]
  Plan 2/1(accelOut) -> [OUT21]
  Plan 2/2(conditionCheckOut) -> [OUT22]
  Plan 2/3(commandAngleOut) -> [OUT23]
  Plan 2/4(planStatusOut) -> [OUT24]
  Plan 2/5(ACCTriggerOut) -> [OUT25]
  [OUT11] -> Multiport Switch/2
  [OUT21] -> Multiport Switch/3
  [OUT12] -> Multiport Switch1/2
  [OUT22] -> Multiport Switch1/3
  [OUT13] -> Multiport Switch2/2
  [OUT23] -> Multiport Switch2/3
  [OUT14] -> Multiport Switch3/2
  [OUT24] -> Multiport Switch3/3
  [OUT15] -> Multiport Switch4/2
  [OUT25] -> Multiport Switch4/3

== system mOvertakeManeuver/Smart Actor/Smart Actor system/Planner/Plan selector ==
  selectNewPlan : TriggerPort  TriggerType=function-call  IsSimulinkFunction=on  FunctionName=selectNewPlan  FunctionVisibility=scoped  VariantControl=(inherit)
  Choose plan : MATLAB Function  TreatAsAtomicUnit=on
  egoState : ArgIn  OutDataTypeStr=Bus: Vehicle  ArgumentName=currPose
  planID : ArgOut  DisableCoverage=on  ArgumentName=planID
  wires:
  Choose plan/1(planId) -> planID/1
  egoState/1 -> Choose plan/1(currPose)

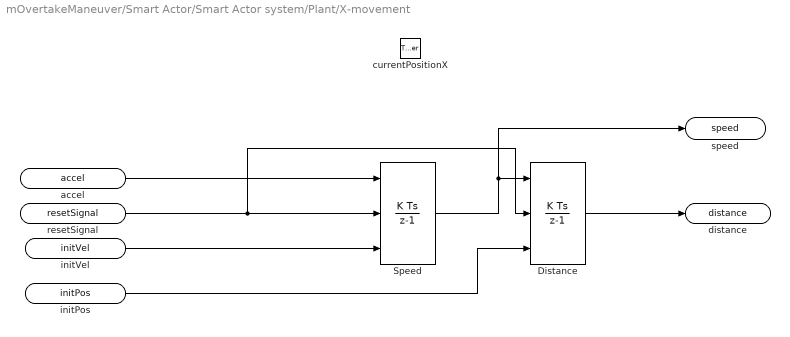
== system mOvertakeManeuver/Smart Actor/Smart Actor system/Plant/X-movement ==
  currentPositionX : TriggerPort  TriggerType=function-call  IsSimulinkFunction=on  FunctionName=currentPositionX  FunctionVisibility=scoped  VariantControl=(inherit)
  Distance : DiscreteIntegrator  ExternalReset=level  InitialConditionSource=external  SampleTime=-1  ICPrevOutput=DiscIntNeverNeededParam  ICPrevScaledInput=DiscIntNeverNeededParam
  Speed : DiscreteIntegrator  ExternalReset=level  InitialConditionSource=external  SampleTime=-1  ICPrevOutput=DiscIntNeverNeededParam  ICPrevScaledInput=DiscIntNeverNeededParam
  accel : ArgIn  ArgumentName=accel
  resetSignal : ArgIn  Port=2  ArgumentName=resetSignal
  initVel : ArgIn  Port=3  ArgumentName=initVel
  initPos : ArgIn  Port=4  ArgumentName=initPos
  distance : ArgOut  ArgumentName=distance
  speed : ArgOut  Port=2  ArgumentName=speed
  wires:
  initPos/1 -> Distance/3
  Speed/1 -> Distance/1, speed/1
  Distance/1 -> distance/1
  accel/1 -> Speed/1
  resetSignal/1 -> Distance/2, Speed/2
  initVel/1 -> Speed/3

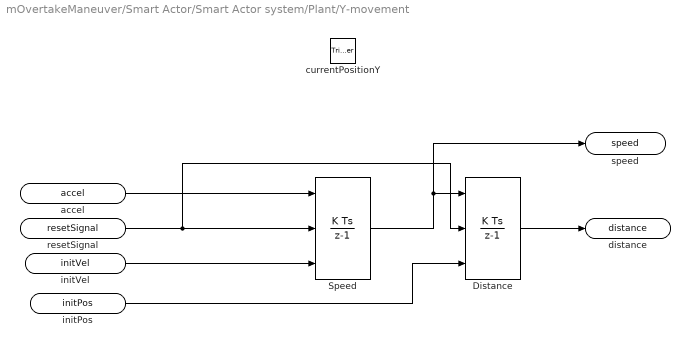
== system mOvertakeManeuver/Smart Actor/Smart Actor system/Plant/Y-movement ==
  currentPositionY : TriggerPort  TriggerType=function-call  IsSimulinkFunction=on  FunctionName=currentPositionY  FunctionVisibility=scoped  VariantControl=(inherit)
  Distance : DiscreteIntegrator  ExternalReset=level  InitialConditionSource=external  SampleTime=-1  ICPrevOutput=DiscIntNeverNeededParam  ICPrevScaledInput=DiscIntNeverNeededParam
  Speed : DiscreteIntegrator  ExternalReset=level  InitialConditionSource=external  SampleTime=-1  ICPrevOutput=DiscIntNeverNeededParam  ICPrevScaledInput=DiscIntNeverNeededParam
  accel : ArgIn  ArgumentName=accel
  resetSignal : ArgIn  Port=2  ArgumentName=resetSignal
  initVel : ArgIn  Port=3  ArgumentName=initVel
  initPos : ArgIn  Port=4  ArgumentName=initPos
  distance : ArgOut  ArgumentName=distance
  speed : ArgOut  Port=2  ArgumentName=speed
  wires:
  initVel/1 -> Speed/3
  initPos/1 -> Distance/3
  Distance/1 -> distance/1
  Speed/1 -> Distance/1, speed/1
  accel/1 -> Speed/1
  resetSignal/1 -> Distance/2, Speed/2

== system mOvertakeManeuver/Wiedemann-74 Driver Model/Apply driver-model/Calculate updated Poses based on driver model/Update Poses ==
  accVector : Inport
  initVelVector : Inport  Port=2
  initPosVector : Inport  Port=3
  Constant : Constant  Value=0
  Discrete-Time Integrator : DiscreteIntegrator  ExternalReset=level  InitialConditionSource=external  SampleTime=-1  ICPrevOutput=DiscIntNeverNeededParam  ICPrevScaledInput=DiscIntNeverNeededParam
  Discrete-Time Integrator1 : DiscreteIntegrator  ExternalReset=level  InitialConditionSource=external  SampleTime=-1  ICPrevOutput=DiscIntNeverNeededParam  ICPrevScaledInput=DiscIntNeverNeededParam
  Out1 : Outport
  Out2 : Outport  Port=2
  wires:
  Discrete-Time Integrator/1 -> Discrete-Time Integrator1/1, Out1/1
  initVelVector/1 -> Discrete-Time Integrator/3
  accVector/1 -> Discrete-Time Integrator/1
  Discrete-Time Integrator1/1 -> Out2/1
  initPosVector/1 -> Discrete-Time Integrator1/3
  Constant/1 -> Discrete-Time Integrator1/2, Discrete-Time Integrator/2

== system mOvertakeManeuver/Wiedemann-74 Driver Model/Apply driver-model/Wiedemann-driver-model/Apply Transfer Function ==
  egoAccCmd : Inport  Partition=on  PartitionDimension=1  PartitionWidth=1  PartitionOffset=0
  Discrete Transfer Fcn : DiscreteTransferFcn  Denominator=[1 0.05]
  For Each : ForEach  DisableCoverage=on  IndexMode=One-based
  Out1 : Outport  ConcatenationDimension=1
  wires:
  egoAccCmd/1 -> Discrete Transfer Fcn/1
  Discrete Transfer Fcn/1 -> Out1/1

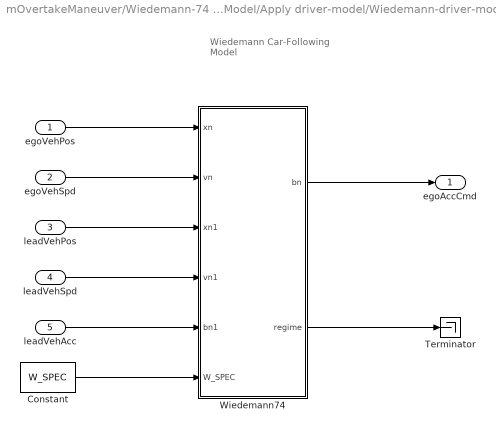
== system mOvertakeManeuver/Wiedemann-74 Driver Model/Apply driver-model/Wiedemann-driver-model/Judgement ==
  note: Wiedemann
      | Car-Following Model
  egoVehPos : Inport
  egoVehSpd : Inport  Port=2
  leadVehPos : Inport  Port=3
  leadVehSpd : Inport  Port=4
  leadVehAcc : Inport  Port=5
  Constant : Constant  Value=W_SPEC  SampleTime=-1
  Terminator : Terminator
  Wiedemann74 : MATLAB Function  TreatAsAtomicUnit=on
  egoAccCmd : Outport
  wires:
  Constant/1 -> Wiedemann74/6(W_SPEC)
  Wiedemann74/1(bn) -> egoAccCmd/1
  Wiedemann74/2(regime) -> Terminator/1
  leadVehAcc/1 -> Wiedemann74/5(bn1)
  leadVehSpd/1 -> Wiedemann74/4(vn1)
  egoVehPos/1 -> Wiedemann74/1(xn)
  leadVehPos/1 -> Wiedemann74/3(xn1)
  egoVehSpd/1 -> Wiedemann74/2(vn)

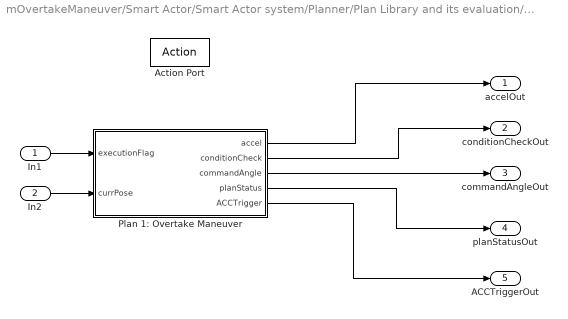
== system mOvertakeManeuver/Smart Actor/Smart Actor system/Planner/Plan Library and its evaluation/Plan 1 ==
  In1 : Inport
  In2 : Inport  Port=2  OutDataTypeStr=Bus: Vehicle
  Action Port : ActionPort  ActionType=case
  Plan 1: Overtake Maneuver : Stateflow chart  TreatAsAtomicUnit=on
  accelOut : Outport
  conditionCheckOut : Outport  Port=2
  commandAngleOut : Outport  Port=3
  planStatusOut : Outport  Port=4
  ACCTriggerOut : Outport  Port=5
  wires:
  Plan 1: Overtake Maneuver/4(planStatus) -> planStatusOut/1
  Plan 1: Overtake Maneuver/5(ACCTrigger) -> ACCTriggerOut/1
  Plan 1: Overtake Maneuver/2(conditionCheck) -> conditionCheckOut/1
  Plan 1: Overtake Maneuver/3(commandAngle) -> commandAngleOut/1
  Plan 1: Overtake Maneuver/1(accel) -> accelOut/1
  In1/1 -> Plan 1: Overtake Maneuver/1(executionFlag)
  In2/1 -> Plan 1: Overtake Maneuver/2(currPose)

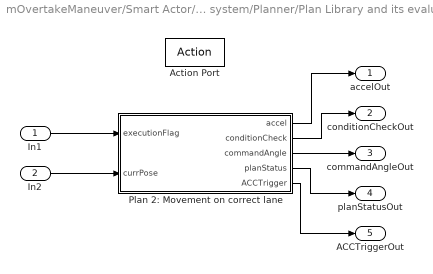
== system mOvertakeManeuver/Smart Actor/Smart Actor system/Planner/Plan Library and its evaluation/Plan 2 ==
  In1 : Inport
  In2 : Inport  Port=2
  Action Port : ActionPort  ActionType=case
  Plan 2: Movement on correct lane : Stateflow chart  TreatAsAtomicUnit=on
  accelOut : Outport
  conditionCheckOut : Outport  Port=2
  commandAngleOut : Outport  Port=3
  planStatusOut : Outport  Port=4
  ACCTriggerOut : Outport  Port=5
  wires:
  In1/1 -> Plan 2: Movement on correct lane/1(executionFlag)
  In2/1 -> Plan 2: Movement on correct lane/2(currPose)
  Plan 2: Movement on correct lane/1(accel) -> accelOut/1
  Plan 2: Movement on correct lane/3(commandAngle) -> commandAngleOut/1
  Plan 2: Movement on correct lane/2(conditionCheck) -> conditionCheckOut/1
  Plan 2: Movement on correct lane/4(planStatus) -> planStatusOut/1
  Plan 2: Movement on correct lane/5(ACCTrigger) -> ACCTriggerOut/1

== system mOvertakeManeuver/Smart Actor/Smart Actor system/Planner/Plan Library and its evaluation/Plan 1/Plan 1: Overtake Maneuver/checkOvertakeFeasibility ==
  currPose : Inport  OutDataTypeStr=Bus: Vehicle  PortDimensions=1
  f : TriggerPort  TriggerType=function-call  VariantControl=(inherit)
      settings: CopyFcn=Stateflow.SLINSF.SimulinkMan.removeBlockPreDeleteFcn  PreDeleteFcn=Stateflow.SLINSF.SimulinkMan.unsafePredeleteFcn
  Check feasibilty of the overtake : Stateflow chart  TreatAsAtomicUnit=on
  feasibilityFlag : Outport
  timeOppLane : Outport  Port=2
  wires:
  Check feasibilty of the overtake/2(t2) -> timeOppLane/1
  Check feasibilty of the overtake/1(overtakeDecision) -> feasibilityFlag/1
  currPose/1 -> Check feasibilty of the overtake/1(currPose)

== matlab function mOvertakeManeuver/Services/Find vehicles ahead in the same lane/MATLAB Function ==
  data: refPose input; matched output; candidatePose input; sensorRange parameter; numLanes parameter
function matched = findVehiclesAheadSameLane(refPose, candidatePose, sensorRange, numLanes)
% For any vehicle, get the vehicles ahead in the same lane.Query is assumed
% to called for a vehicle moving in +ve x-direction.
% refPose - Query-Calling vehicle
% candidatePose - Actor to be processed as candidate for matching the query criteria.

laneBoundaries = zeros(1, numLanes + 1);
% Getting the key corresponding to the actorId from data-table
key = getScenarioTableEntryKey(uint32(1), refPose.ActorID);
completeLaneBoundaryInfo = getScenarioTableEntry(key);
for i = 1 : size(laneBoundaries, 2)
    laneBoundaries(1, i) = completeLaneBoundaryInfo.coordinates(i, 2);
end
laneIndx = -1;

if refPose.Yaw == 0
    vehicleDirection = 1; % +1 means positive - x
elseif refPose.Yaw == 180
    vehicleDirection = -1; % -1 means negative - x
else
    vehicleDirection = 0;
end

% Find own lane information based on lane boundary info and own position.
for i = 1 : size(laneBoundaries, 2) - 1
    if (refPose.Position(2) <= laneBoundaries(1, i) && refPose.Position(2) >= laneBoundaries(1, (i + 1)))
        laneIndx = i;
        break;
    elseif (refPose.Position(2) >= laneBoundaries(1, i) && refPose.Position(2) <= laneBoundaries(1, (i + 1)))
        laneIndx = i;
        break;
    end
end

if laneIndx < 0
    matched = false;
elseif laneIndx <= numLanes
    % Candidate actor must be ahead AND in Range AND In same lane
    if vehicleDirection == 1
        if ((candidatePose.Position(1) - refPose.Position(1)) > 0 && ...
                (candidatePose.Position(1) - refPose.Position(1) < sensorRange) && ...
                (candidatePose.Position(2) <= laneBoundaries(1, laneIndx)) && (candidatePose.Position(2) >= laneBoundaries(1, (laneIndx + 1))))
            matched = true;
        else
            matched = false;
        end
    elseif vehicleDirection == -1
        if ((refPose.Position(1) - candidatePose.Position(1)) > 0 && ...
                ((refPose.Position(1) - candidatePose.Position(1)) < sensorRange) && ...
                (candidatePose.Position(2) >= laneBoundaries(1, laneIndx)) && ...
                (candidatePose.Position(2) <= laneBoundaries(1, (laneIndx + 1))))
            matched = true;
        else
            matched = false;
        end
    else
        matched = false;
    end
else
    matched = false;
end
